simulink model "PMSM_Sensorless_ADRC_PI_cmp"  (R2019b)
settings: Solver=VariableStepAuto  StartTime=0.0  StopTime=10.0  RelTol=1e-3
libraries: powerlib x4, simulink x1
settings Model: Creator=李瑾年  LastModifiedBy=李瑾年

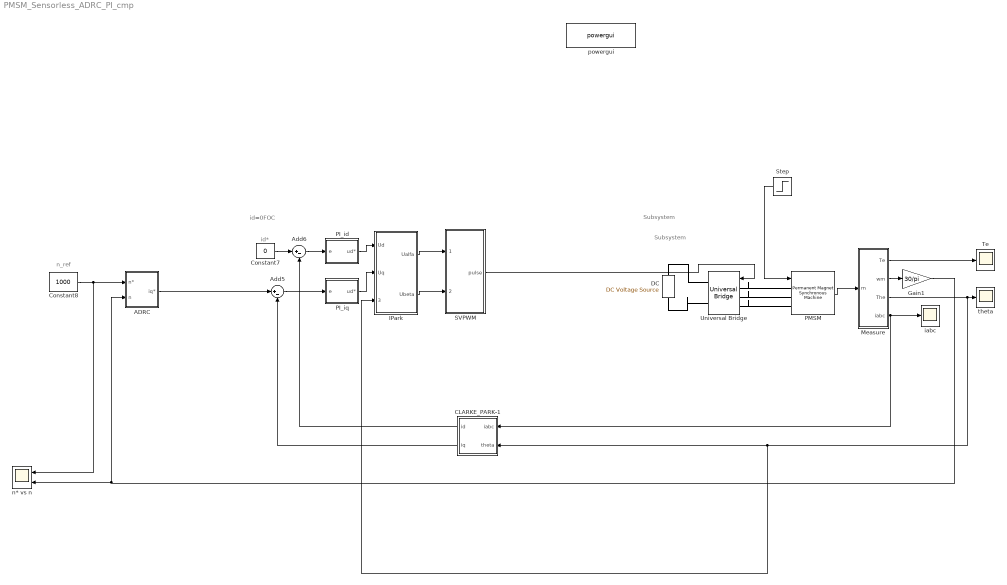
== system PMSM_Sensorless_ADRC_PI_cmp ==
  note: Subsystem
  note: id=0FOC
  note: n_ref
  note: id*
  note: Subsystem
  ADRC : Subsystem
  Add5 : Sum  Inputs=|+-
  Add6 : Sum  Inputs=|+-
  CLARKE_PARK-1 : Subsystem
  Constant7 : Constant  Value=0
  Constant8 : Constant  Value=1000
  DC : powerlib/Electrical Sources/DC Voltage Source  Amplitude=311  Measurements=None
      settings: SourceProductName=Simscape Electrical
  Gain1 : Gain  Gain=30/pi
  IPark : Subsystem
  Measure : Subsystem
  PI_id : Subsystem
      mask Display: disp('PI')
  PI_iq : Subsystem
      mask Display: disp('PI')
  PMSM : powerlib/Machines/Permanent Magnet Synchronous Machine  NbPhases=3  FluxDistribution=Sinusoidal  RotorType=Salient-pole  MechanicalLoad=Torque Tm  PresetModel=No  ShowDetailedParameters=on  MeasurementBus=off  Resistance=2.8750  Inductance=8.5e-3  dqInductances=[8.5e-3, 8.5e-3]  La=0.000835  MachineConstant=Flux linkage established by magnets (V.s)  Flux=0.175  VoltageCst=126.966  TorqueCst=1.05  Flat=120  Mechanical="[ 1e-3, 0,  4 ]"  PolePairs=4  InitialConditions=[0,0, 0,0]  InitialConditions5ph=[0 0 0 0 0 0]  RefAngle=Aligned with phase A axis (original Park)  IterativeDiscreteModel=Trapezoidal non iterative  TsBlock=-1  TsPowergui=0
  SVPWM : Subsystem
  Step : Step  Time=0.2  After=2  SampleTime=0
  Te : Scope
  Universal Bridge : powerlib/Power Electronics/Universal Bridge  Arms=3  SnubberResistance=1e5  SnubberCapacitance=inf  Device=IGBT / Diodes  Ron=1e-3  Lon=0  ForwardVoltages="[  0  0  ]"  ForwardVoltage=0  GTOparameters=[ 10e-6 , 20e-6 ]  IGBTparameters=[ 1e-6 , 2e-6 ]  Measurements=None  Measurements_2=None  converterType=Rectifier
      settings: SourceProductName=Simscape Electrical
  iabc : Scope
  n* vs n : Scope  NumInputPorts=2
  powergui : powerlib/powergui  Priority=1  SimulationMode=Discrete  SampleTime=2e-7  frequency=60  Iterations=50  frequencyindice=0  Pbase=100e6  ErrMax=1e-4  UnitsV=kV  UnitsW=MW  buscounter=0  FunctionMessages=off  echomessages=off  EnableUseOfTLC=off  CurrentSourceSwitches=off  DisableSnubberDevices=off  DisableRonSwitches=off  DisableVfSwitches=off  DisplayEquations=off  AutomaticDiscreteSolvers=off  SolverType=Tustin/Backward Euler (TBE)  Interpol=off  ExternalGateDelay=off  methode=off  Ts=100  x0status=blocks  SPID=off  SwTol=0  HookPort=off  NonlinearTolerance=1e-4  nMaxIteration=100  ContinueOnMaxIteration=off  RestoreLinks=warning  ResistiveCurrentMeasurement=off  Frange=[0:2:500]  Ylog=off  Xlog=on  ShowGrid=off  save=off  variable=ZData  structure=0  ZoomFFT=off  StartTime=0.0  cycles=1  DisplayStyle=1  fundamental=60  FreqAxis=off  MaxFrequency=1000  frequencyindicesteady=1  RmsSteady=1  display=off
      settings: SourceProductName=Simscape Electrical
  theta : Scope
  wires:
  Constant8/1 -> n* vs n/1, ADRC/1(n*)
  ADRC/1(iq*) -> Add5/1
  CLARKE_PARK-1/2(iq) -> Add5/2
  CLARKE_PARK-1/1(id) -> Add6/2
  PI_iq/1(ud*) -> IPark/2(Uq)
  IPark/1(Ualfa) -> SVPWM/1(Valpha)
  Add6/1 -> PI_id/1(e)
  Constant7/1 -> Add6/1
  IPark/2(Ubeta) -> SVPWM/2(Vbeta)
  Add5/1 -> PI_iq/1(e)
  PI_id/1(ud*) -> IPark/1(Ud)
  Gain1/1 -> n* vs n/2, ADRC/2(n)
  Measure/4(iabc) -> CLARKE_PARK-1/1(iabc), iabc/1
  Measure/3(The) -> IPark/3(theta_ADRC), CLARKE_PARK-1/2(theta), theta/1
  SVPWM/1(pulse) -> Universal Bridge/1
  Step/1 -> PMSM/1
  Measure/2(wm) -> Gain1/1
  PMSM/1 -> Measure/1(m)
  Measure/1(Te) -> Te/1
  connections:
  DC/LConn1 -- Universal Bridge/RConn2
  Universal Bridge/LConn3 -- PMSM/LConn3
  Universal Bridge/RConn1 -- DC/RConn1
  Universal Bridge/LConn2 -- PMSM/LConn2
  Universal Bridge/LConn1 -- PMSM/LConn1

== system PMSM_Sensorless_ADRC_PI_cmp/ADRC ==
  n* : Inport
  n : Inport  Port=2
  ESO : Subsystem
  Saturation : Saturate  UpperLimit=12  LowerLimit=-12
  first_order_TD : Subsystem
  nlsef : Subsystem
  iq* : Outport
  wires:
  n/1 -> ESO/2(n)
  nlsef/1(ut) -> Saturation/1, ESO/1(ut)
  ESO/2(z22) -> nlsef/2(z22)
  ESO/1(z21) -> nlsef/3(z21)
  first_order_TD/1(z11) -> nlsef/1(z11)
  n*/1 -> first_order_TD/1(n*)
  Saturation/1 -> iq*/1

== system PMSM_Sensorless_ADRC_PI_cmp/CLARKE_PARK-1 ==
  iabc : Inport
  theta : Inport  Port=2
  Clark1 : Subsystem
  Demux1 : Demux  Outputs=3
  Park1 : Subsystem
  id : Outport
  iq : Outport  Port=2
  wires:
  Park1/2(Q) -> iq/1
  Clark1/1(Alpha) -> Park1/1(Alpha)
  Demux1/1 -> Clark1/1(A)
  Demux1/3 -> Clark1/3(C)
  Demux1/2 -> Clark1/2(B)
  Clark1/2(Beta) -> Park1/2(Beta)
  theta/1 -> Park1/3(The)
  iabc/1 -> Demux1/1
  Park1/1(D) -> id/1

== system PMSM_Sensorless_ADRC_PI_cmp/IPark ==
  Ud : Inport
  Uq : Inport  Port=2
  theta_ADRC : Inport  Port=3
  Fcn : Fcn  Expr=cos(u[3])*u[2]-sin(u[3])*u[1]
  Fcn1 : Fcn  Expr=sin(u[3])*u[2]+cos(u[3])*u[1]
  Mux : Mux  Inputs=3
  Ualfa : Outport
  Ubeta : Outport  Port=2
  wires:
  Uq/1 -> Mux/1
  Ud/1 -> Mux/2
  theta_ADRC/1 -> Mux/3
  Mux/1 -> Fcn/1, Fcn1/1
  Fcn/1 -> Ualfa/1
  Fcn1/1 -> Ubeta/1

== system PMSM_Sensorless_ADRC_PI_cmp/Measure ==
  note: P
  m : Inport
  Bus Creator : BusCreator  Inputs=3
  Bus Selector1 : BusSelector  OutputSignals=Rotor speed wm (rad/s),Rotor angle thetam (rad),Electromagnetic torque Te (N*m),Stator current is_a (A),Stator current is_b (A),Stator current is_c (A)
  Constant5 : Constant  Value=2*pi
  Gain2 : Gain  Gain=4
  Math Function1 : Math  Operator=mod  SaturateOnIntegerOverflow=on
  Te : Outport
  wm : Outport  Port=2
  The : Outport  Port=3
  iabc : Outport  Port=4
  wires:
  Bus Selector1/2 -> Gain2/1  "<Rotor angle thetam (rad)>"
  Bus Selector1/3 -> Te/1  "<Electromagnetic torque Te (N*m)>"
  m/1 -> Bus Selector1/1
  Bus Selector1/1 -> wm/1  "<Rotor speed wm (rad/s)>"
  Bus Selector1/6 -> Bus Creator/3  "<Stator current is_c (A)>"
  Bus Selector1/5 -> Bus Creator/2  "<Stator current is_b (A)>"
  Bus Selector1/4 -> Bus Creator/1  "<Stator current is_a (A)>"
  Bus Creator/1 -> iabc/1
  Gain2/1 -> Math Function1/1
  Constant5/1 -> Math Function1/2
  Math Function1/1 -> The/1

== system PMSM_Sensorless_ADRC_PI_cmp/PI_id ==
  e : Inport
  Add : Sum
  Integrator : Integrator
  Ki=R*500 : Gain  Gain=2.875*100
  Kp=L*3000 : Gain  Gain=8.5e-3*2000
  Saturation : Saturate  UpperLimit=250  LowerLimit=-250
  ud* : Outport
  wires:
  Ki=R*500/1 -> Integrator/1
  e/1 -> Kp=L*3000/1, Ki=R*500/1
  Saturation/1 -> ud*/1
  Integrator/1 -> Add/2
  Kp=L*3000/1 -> Add/1
  Add/1 -> Saturation/1

== system PMSM_Sensorless_ADRC_PI_cmp/PI_iq ==
  e : Inport
  Add : Sum
  Integrator : Integrator
  Ki=R*500 : Gain  Gain=2.875*100
  Kp=L*3000 : Gain  Gain=8.5e-3*2000
  Saturation : Saturate  UpperLimit=250  LowerLimit=-250
  ud* : Outport
  wires:
  Ki=R*500/1 -> Integrator/1
  e/1 -> Kp=L*3000/1, Ki=R*500/1
  Saturation/1 -> ud*/1
  Integrator/1 -> Add/2
  Kp=L*3000/1 -> Add/1
  Add/1 -> Saturation/1

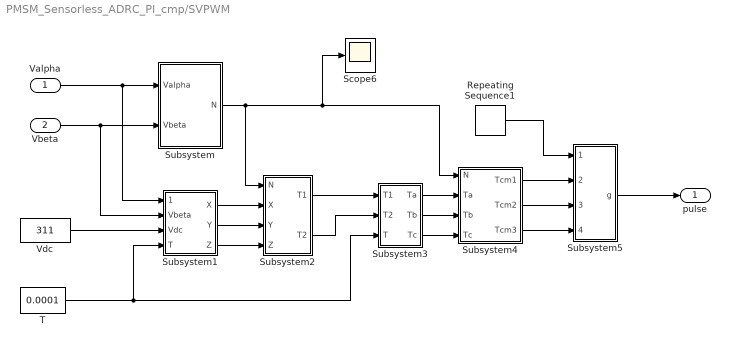
== system PMSM_Sensorless_ADRC_PI_cmp/SVPWM ==
  Valpha : Inport
  Vbeta : Inport  Port=2
  Repeating Sequence1 : simulink/Sources/Repeating Sequence  rep_seq_t=[0 0.00005 0.0001]  rep_seq_y=[0 0.00005 0]
  Scope6 : Scope
  Subsystem : Subsystem
  Subsystem1 : Subsystem
  Subsystem2 : Subsystem
  Subsystem3 : Subsystem
  Subsystem4 : Subsystem
  Subsystem5 : Subsystem
  T : Constant  Value=0.0001
  Vdc : Constant  Value=311
  pulse : Outport
  wires:
  Subsystem5/1(g) -> pulse/1
  Repeating Sequence1/1 -> Subsystem5/1(Carrier)
  Subsystem4/3(Tcm3) -> Subsystem5/4(Tcm3)
  Subsystem4/2(Tcm2) -> Subsystem5/3(Tcm2)
  Subsystem4/1(Tcm1) -> Subsystem5/2(Tcm1)
  Subsystem3/3(Tc) -> Subsystem4/4(Tc)
  Subsystem3/2(Tb) -> Subsystem4/3(Tb)
  Subsystem3/1(Ta) -> Subsystem4/2(Ta)
  Subsystem2/2(T2) -> Subsystem3/2(T2)
  Subsystem2/1(T1) -> Subsystem3/1(T1)
  Subsystem1/3(Z) -> Subsystem2/4(Z)
  Subsystem1/2(Y) -> Subsystem2/3(Y)
  Subsystem1/1(X) -> Subsystem2/2(X)
  Subsystem/1(N) -> Subsystem2/1(N), Scope6/1, Subsystem4/1(N)
  Vdc/1 -> Subsystem1/3(Vdc)
  T/1 -> Subsystem3/3(T), Subsystem1/4(T)
  Vbeta/1 -> Subsystem1/2(Vbeta), Subsystem/2(Vbeta)
  Valpha/1 -> Subsystem1/1(Valpha), Subsystem/1(Valpha)

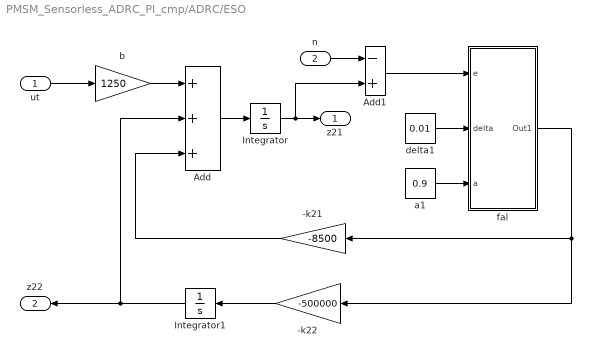
== system PMSM_Sensorless_ADRC_PI_cmp/ADRC/ESO ==
  ut : Inport
  n : Inport  Port=2
  -k21 : Gain  Gain=-8500
  -k22 : Gain  Gain=-500000
  Add : Sum  Inputs=+++
  Add1 : Sum  Inputs=-+
  Integrator : Integrator
  Integrator1 : Integrator
  a1 : Constant  Value=0.9
  b : Gain  Gain=1250
  delta1 : Constant  Value=0.01
  fal : Subsystem
  z21 : Outport
  z22 : Outport  Port=2
  wires:
  ut/1 -> b/1
  b/1 -> Add/1
  Add/1 -> Integrator/1
  Integrator/1 -> z21/1, Add1/2
  n/1 -> Add1/1
  Add1/1 -> fal/1(e)
  delta1/1 -> fal/2(delta)
  a1/1 -> fal/3(a)
  fal/1(Out1) -> -k21/1, -k22/1
  -k21/1 -> Add/3
  -k22/1 -> Integrator1/1
  Integrator1/1 -> Add/2, z22/1

== system PMSM_Sensorless_ADRC_PI_cmp/ADRC/first_order_TD ==
  n* : Inport
  -k0 : Gain  Gain=-6500
  Add : Sum  Inputs=-+
  Integrator : Integrator
  a0 : Constant  Value=0.4
  delta0 : Constant  Value=0.01
  fal : Subsystem
  z11 : Outport
  wires:
  Add/1 -> fal/1(e)
  delta0/1 -> fal/2(delta)
  a0/1 -> fal/3(a)
  fal/1(Out1) -> -k0/1
  -k0/1 -> Integrator/1
  Integrator/1 -> Add/2, z11/1
  n*/1 -> Add/1

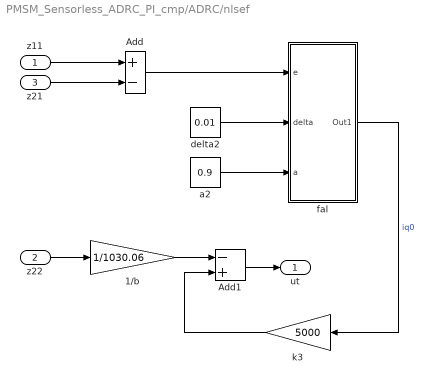
== system PMSM_Sensorless_ADRC_PI_cmp/ADRC/nlsef ==
  z11 : Inport
  z22 : Inport  Port=2
  z21 : Inport  Port=3
  1/b : Gain  Gain=1/1030.06
  Add : Sum  Inputs=+-
  Add1 : Sum  Inputs=-+
  a2 : Constant  Value=0.9
  delta2 : Constant  Value=0.01
  fal : Subsystem
  k3 : Gain  Gain=5000
  ut : Outport
  wires:
  z11/1 -> Add/1
  z21/1 -> Add/2
  Add/1 -> fal/1(e)
  delta2/1 -> fal/2(delta)
  a2/1 -> fal/3(a)
  fal/1(Out1) -> k3/1  "iq0"
  z22/1 -> 1/b/1
  Add1/1 -> ut/1
  k3/1 -> Add1/2
  1/b/1 -> Add1/1

== system PMSM_Sensorless_ADRC_PI_cmp/CLARKE_PARK-1/Clark1 ==
  A : Inport
  B : Inport  Port=2
  C : Inport  Port=3
  Mux : Mux  Inputs=3
  alpha : Fcn  Expr=(u(1)-0.5*(u(2)+u(3)))*2/3
  beta : Fcn  Expr=sqrt(3)/2*(u(2)-u(3))*2/3
  Alpha : Outport
  Beta : Outport  Port=2
  wires:
  beta/1 -> Beta/1
  Mux/1 -> alpha/1, beta/1
  A/1 -> Mux/1
  C/1 -> Mux/3
  B/1 -> Mux/2
  alpha/1 -> Alpha/1

== system PMSM_Sensorless_ADRC_PI_cmp/CLARKE_PARK-1/Park1 ==
  Alpha : Inport
  Beta : Inport  Port=2
  The : Inport  Port=3
  Mux : Mux  Inputs=3
  d : Fcn  Expr=u(1)*cos(u(3))+u(2)*sin(u(3))
  q : Fcn  Expr=-u(1)*sin(u(3))+u(2)*cos(u(3))
  D : Outport
  Q : Outport  Port=2
  wires:
  The/1 -> Mux/3
  q/1 -> Q/1
  Mux/1 -> d/1, q/1
  Alpha/1 -> Mux/1
  Beta/1 -> Mux/2
  d/1 -> D/1

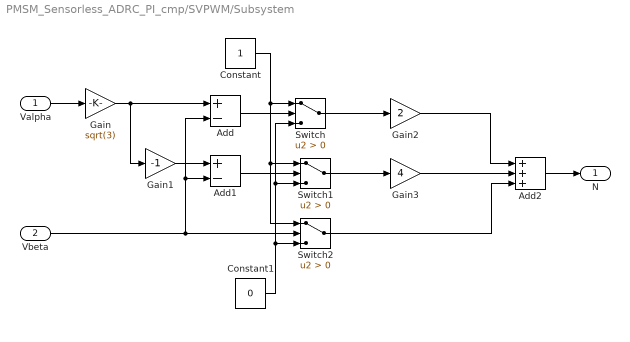
== system PMSM_Sensorless_ADRC_PI_cmp/SVPWM/Subsystem ==
  Valpha : Inport
  Vbeta : Inport  Port=2
  Add : Sum  Inputs=+-
  Add1 : Sum  Inputs=+-
  Add2 : Sum  Inputs=+++
  Constant : Constant
  Constant1 : Constant  Value=0
  Gain : Gain  Gain=sqrt(3)
  Gain1 : Gain  Gain=-1
  Gain2 : Gain  Gain=2
  Gain3 : Gain  Gain=4
  Switch : Switch  Criteria=u2 > Threshold
  Switch1 : Switch  Criteria=u2 > Threshold
  Switch2 : Switch  Criteria=u2 > Threshold
  N : Outport
  wires:
  Valpha/1 -> Gain/1
  Gain3/1 -> Add2/2
  Gain2/1 -> Add2/1
  Add1/1 -> Switch1/2
  Gain1/1 -> Add1/1
  Switch1/1 -> Gain3/1
  Switch2/1 -> Add2/3
  Switch/1 -> Gain2/1
  Add/1 -> Switch/2
  Gain/1 -> Gain1/1, Add/1
  Constant1/1 -> Switch/3, Switch1/3, Switch2/3
  Constant/1 -> Switch1/1, Switch2/1, Switch/1
  Vbeta/1 -> Add1/2, Add/2, Switch2/2
  Add2/1 -> N/1

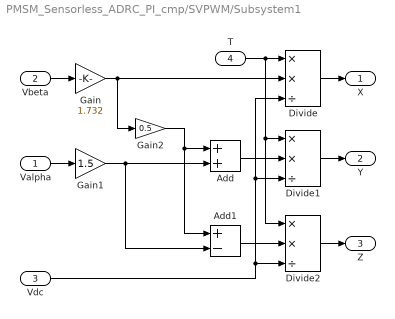
== system PMSM_Sensorless_ADRC_PI_cmp/SVPWM/Subsystem1 ==
  Valpha : Inport
  Vbeta : Inport  Port=2
  Vdc : Inport  Port=3
  T : Inport  Port=4
  Add : Sum
  Add1 : Sum  Inputs=+-
  Divide : Product  Inputs=**/
  Divide1 : Product  Inputs=**/
  Divide2 : Product  Inputs=**/
  Gain : Gain  Gain=1.732
  Gain1 : Gain  Gain=1.5
  Gain2 : Gain  Gain=0.5
  X : Outport
  Y : Outport  Port=2
  Z : Outport  Port=3
  wires:
  Divide2/1 -> Z/1
  Divide1/1 -> Y/1
  Divide/1 -> X/1
  Valpha/1 -> Gain1/1
  Vbeta/1 -> Gain/1
  Add1/1 -> Divide2/2
  Add/1 -> Divide1/2
  Gain1/1 -> Add1/2, Add/2
  Gain2/1 -> Add/1, Add1/1
  Gain/1 -> Divide/2, Gain2/1
  Vdc/1 -> Divide/3, Divide1/3, Divide2/3
  T/1 -> Divide2/1, Divide1/1, Divide/1

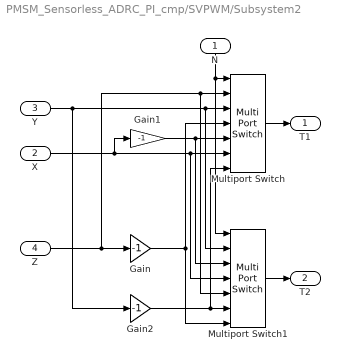
== system PMSM_Sensorless_ADRC_PI_cmp/SVPWM/Subsystem2 ==
  N : Inport
  X : Inport  Port=2
  Y : Inport  Port=3
  Z : Inport  Port=4
  Gain : Gain  Gain=-1
  Gain1 : Gain  Gain=-1
  Gain2 : Gain  Gain=-1
  Multiport Switch : MultiPortSwitch  Inputs=6  DiagnosticForDefault=None
  Multiport Switch1 : MultiPortSwitch  Inputs=6  DiagnosticForDefault=None
  T1 : Outport
  T2 : Outport  Port=2
  wires:
  Multiport Switch1/1 -> T2/1
  Multiport Switch/1 -> T1/1
  Gain2/1 -> Multiport Switch/7, Multiport Switch1/6
  Gain1/1 -> Multiport Switch1/3, Multiport Switch/5
  X/1 -> Multiport Switch/6, Multiport Switch1/4, Gain1/1
  Gain/1 -> Multiport Switch1/7, Multiport Switch/4
  Y/1 -> Gain2/1, Multiport Switch1/2, Multiport Switch/3
  Z/1 -> Gain/1, Multiport Switch/2, Multiport Switch1/5
  N/1 -> Multiport Switch/1, Multiport Switch1/1

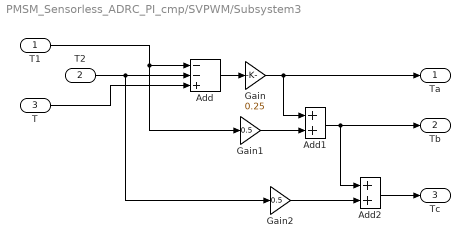
== system PMSM_Sensorless_ADRC_PI_cmp/SVPWM/Subsystem3 ==
  T1 : Inport
  T2 : Inport  Port=2
  T : Inport  Port=3
  Add : Sum  Inputs=--+
  Add1 : Sum
  Add2 : Sum
  Gain : Gain  Gain=0.25
  Gain1 : Gain  Gain=0.5
  Gain2 : Gain  Gain=0.5
  Ta : Outport
  Tb : Outport  Port=2
  Tc : Outport  Port=3
  wires:
  T/1 -> Add/3
  Add2/1 -> Tc/1
  Gain2/1 -> Add2/2
  Add1/1 -> Add2/1, Tb/1
  Gain1/1 -> Add1/2
  Gain/1 -> Add1/1, Ta/1
  Add/1 -> Gain/1
  T2/1 -> Gain2/1, Add/2
  T1/1 -> Add/1, Gain1/1

== system PMSM_Sensorless_ADRC_PI_cmp/SVPWM/Subsystem4 ==
  N : Inport
  Ta : Inport  Port=2
  Tb : Inport  Port=3
  Tc : Inport  Port=4
  Multiport Switch : MultiPortSwitch  Inputs=6  DiagnosticForDefault=None
  Multiport Switch1 : MultiPortSwitch  Inputs=6  DiagnosticForDefault=None
  Multiport Switch2 : MultiPortSwitch  Inputs=6  DiagnosticForDefault=None
  Tcm1 : Outport
  Tcm2 : Outport  Port=2
  Tcm3 : Outport  Port=3
  wires:
  Multiport Switch2/1 -> Tcm3/1
  Multiport Switch1/1 -> Tcm2/1
  Multiport Switch/1 -> Tcm1/1
  N/1 -> Multiport Switch2/1, Multiport Switch1/1, Multiport Switch/1
  Tc/1 -> Multiport Switch1/3, Multiport Switch/6, Multiport Switch/5, Multiport Switch1/7, Multiport Switch2/2, Multiport Switch2/4
  Ta/1 -> Multiport Switch/4, Multiport Switch/3, Multiport Switch1/2, Multiport Switch1/6, Multiport Switch2/5, Multiport Switch2/7
  Tb/1 -> Multiport Switch/2, Multiport Switch/7, Multiport Switch1/4, Multiport Switch1/5, Multiport Switch2/3, Multiport Switch2/6

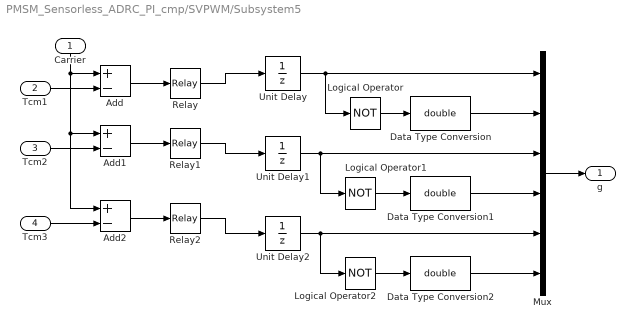
== system PMSM_Sensorless_ADRC_PI_cmp/SVPWM/Subsystem5 ==
  Carrier : Inport
  Tcm1 : Inport  Port=2
  Tcm2 : Inport  Port=3
  Tcm3 : Inport  Port=4
  Add : Sum  Inputs=+-
  Add1 : Sum  Inputs=+-
  Add2 : Sum  Inputs=+-
  Data Type Conversion : DataTypeConversion  OutDataTypeStr=double
  Data Type Conversion1 : DataTypeConversion  OutDataTypeStr=double
  Data Type Conversion2 : DataTypeConversion  OutDataTypeStr=double
  Logical Operator : Logic  Operator=NOT  AllPortsSameDT=off  OutDataTypeStr=boolean
  Logical Operator1 : Logic  Operator=NOT  AllPortsSameDT=off  OutDataTypeStr=boolean
  Logical Operator2 : Logic  Operator=NOT  AllPortsSameDT=off  OutDataTypeStr=boolean
  Mux : Mux  Inputs=6
  Relay : Relay  OffSwitchValue=-eps
  Relay1 : Relay  OffSwitchValue=-eps
  Relay2 : Relay  OffSwitchValue=-eps
  Unit Delay : UnitDelay  SampleTime=-1  HasFrameUpgradeWarning=on
  Unit Delay1 : UnitDelay  SampleTime=-1  HasFrameUpgradeWarning=on
  Unit Delay2 : UnitDelay  SampleTime=-1  HasFrameUpgradeWarning=on
  g : Outport
  wires:
  Tcm3/1 -> Add2/2
  Tcm2/1 -> Add1/2
  Tcm1/1 -> Add/2
  Relay2/1 -> Unit Delay2/1
  Relay1/1 -> Unit Delay1/1
  Relay/1 -> Unit Delay/1
  Unit Delay2/1 -> Mux/5, Logical Operator2/1
  Unit Delay1/1 -> Mux/3, Logical Operator1/1
  Unit Delay/1 -> Logical Operator/1, Mux/1
  Mux/1 -> g/1
  Data Type Conversion/1 -> Mux/2
  Data Type Conversion1/1 -> Mux/4
  Data Type Conversion2/1 -> Mux/6
  Logical Operator2/1 -> Data Type Conversion2/1
  Logical Operator1/1 -> Data Type Conversion1/1
  Logical Operator/1 -> Data Type Conversion/1
  Add1/1 -> Relay1/1
  Add2/1 -> Relay2/1
  Add/1 -> Relay/1
  Carrier/1 -> Add/1, Add2/1, Add1/1

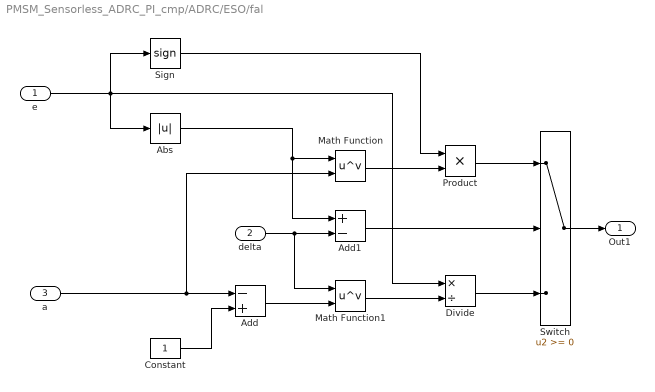
== system PMSM_Sensorless_ADRC_PI_cmp/ADRC/ESO/fal ==
  e : Inport
  delta : Inport  Port=2
  a : Inport  Port=3
  Abs : Abs
  Add : Sum  Inputs=-+
  Add1 : Sum  Inputs=+-
  Constant : Constant
  Divide : Product  Inputs=*/
  Math Function : Math  Operator=pow  SaturateOnIntegerOverflow=on
  Math Function1 : Math  Operator=pow  SaturateOnIntegerOverflow=on
  Product : Product  RndMeth=Zero
  Sign : Signum
  Switch : Switch
  Out1 : Outport
  wires:
  a/1 -> Math Function/2, Add/1
  Constant/1 -> Add/2
  Abs/1 -> Math Function/1, Add1/1
  Math Function/1 -> Product/2
  Sign/1 -> Product/1
  delta/1 -> Add1/2, Math Function1/1
  Add1/1 -> Switch/2
  Product/1 -> Switch/1
  Add/1 -> Math Function1/2
  Math Function1/1 -> Divide/2
  Divide/1 -> Switch/3
  Switch/1 -> Out1/1
  e/1 -> Sign/1, Abs/1, Divide/1

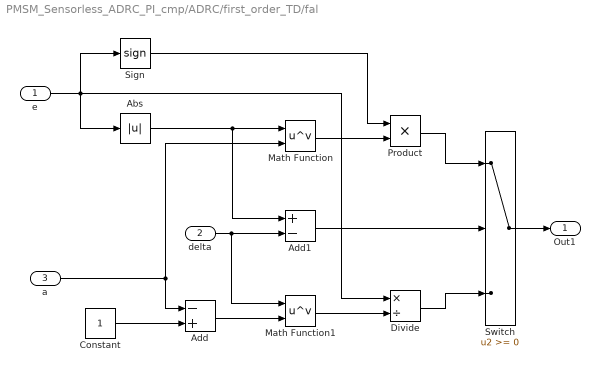
== system PMSM_Sensorless_ADRC_PI_cmp/ADRC/first_order_TD/fal ==
  e : Inport
  delta : Inport  Port=2
  a : Inport  Port=3
  Abs : Abs
  Add : Sum  Inputs=-+
  Add1 : Sum  Inputs=+-
  Constant : Constant
  Divide : Product  Inputs=*/
  Math Function : Math  Operator=pow  SaturateOnIntegerOverflow=on
  Math Function1 : Math  Operator=pow  SaturateOnIntegerOverflow=on
  Product : Product  RndMeth=Zero
  Sign : Signum
  Switch : Switch
  Out1 : Outport
  wires:
  a/1 -> Add/1, Math Function/2
  Constant/1 -> Add/2
  Abs/1 -> Math Function/1, Add1/1
  Math Function/1 -> Product/2
  Sign/1 -> Product/1
  delta/1 -> Add1/2, Math Function1/1
  Add1/1 -> Switch/2
  Product/1 -> Switch/1
  Add/1 -> Math Function1/2
  Math Function1/1 -> Divide/2
  Divide/1 -> Switch/3
  Switch/1 -> Out1/1
  e/1 -> Sign/1, Abs/1, Divide/1

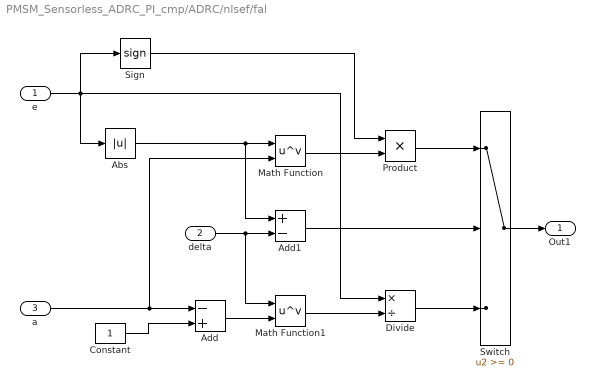
== system PMSM_Sensorless_ADRC_PI_cmp/ADRC/nlsef/fal ==
  e : Inport
  delta : Inport  Port=2
  a : Inport  Port=3
  Abs : Abs
  Add : Sum  Inputs=-+
  Add1 : Sum  Inputs=+-
  Constant : Constant
  Divide : Product  Inputs=*/
  Math Function : Math  Operator=pow  SaturateOnIntegerOverflow=on
  Math Function1 : Math  Operator=pow  SaturateOnIntegerOverflow=on
  Product : Product  RndMeth=Zero
  Sign : Signum
  Switch : Switch
  Out1 : Outport
  wires:
  a/1 -> Math Function/2, Add/1
  Constant/1 -> Add/2
  Abs/1 -> Math Function/1, Add1/1
  Math Function/1 -> Product/2
  Sign/1 -> Product/1
  delta/1 -> Add1/2, Math Function1/1
  Add1/1 -> Switch/2
  Product/1 -> Switch/1
  Add/1 -> Math Function1/2
  Math Function1/1 -> Divide/2
  Divide/1 -> Switch/3
  Switch/1 -> Out1/1
  e/1 -> Sign/1, Abs/1, Divide/1
